simulink model "UnmilsElectrodeMapping"  (R2022b)
settings: Solver=VariableStepAuto  StartTime=0.0  StopTime=10.0  RelTol=1e-3
undefined symbols (not defined in the file or in its folder): ActFx, ActFy, ActFz, ActTx, ActTy, ActTz, dt, max_effort_V, min_effort_V, resolutionV, Ts_V
settings Model: Creator=ryankinzie  LastModifiedBy=ryankinzie

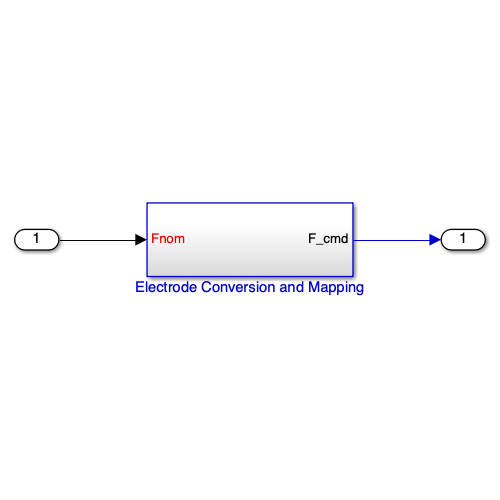
[thumbnail: Simulink's stored preview of the top-level diagram]
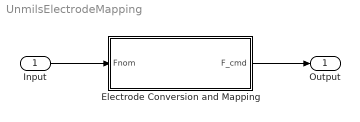
== system UnmilsElectrodeMapping ==
  Input : Inport
  Electrode Conversion and Mapping : Subsystem
  Output : Outport
  wires:
  Input/1 -> Electrode Conversion and Mapping/1(Fnom)
  Electrode Conversion and Mapping/1(F_cmd) -> Output/1

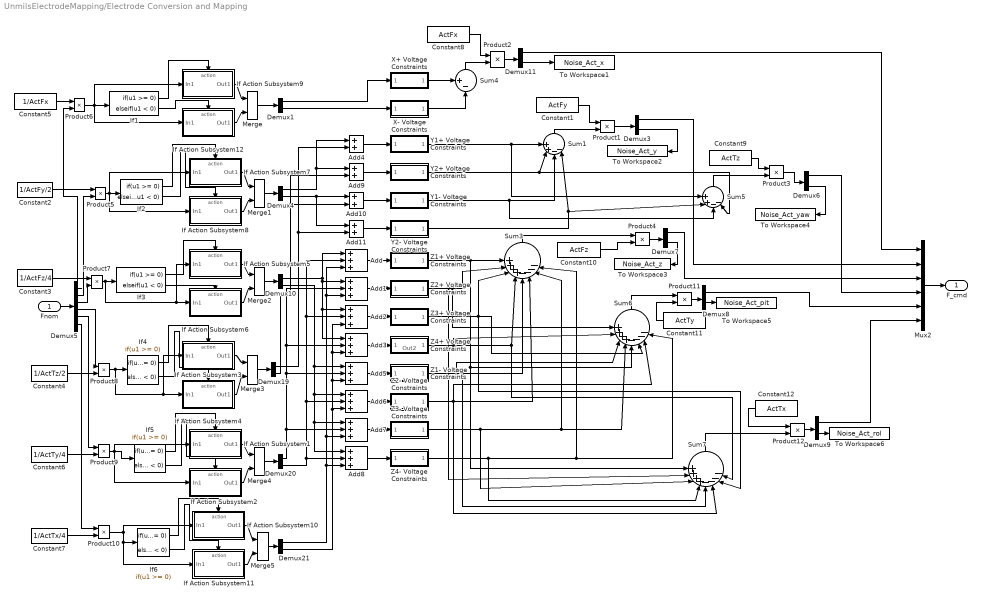
== system UnmilsElectrodeMapping/Electrode Conversion and Mapping ==
  Fnom : Inport
  Add{,1..3,5..8} (8 alike) : Sum  Inputs=+++
  Add{4,9..11} (4 alike) : Sum
  Constant1 : Constant  Value=ActFy
  Constant10 : Constant  Value=ActFz
  Constant11 : Constant  Value=ActTy
  Constant12 : Constant  Value=ActTx
  Constant2 : Constant  Value=1/ActFy/2
  Constant3 : Constant  Value=1/ActFz/4
  Constant4 : Constant  Value=1/ActTz/2
  Constant5 : Constant  Value=1/ActFx
  Constant6 : Constant  Value=1/ActTy/4
  Constant7 : Constant  Value=1/ActTx/4
  Constant8 : Constant  Value=ActFx
  Constant9 : Constant  Value=ActTz
  Demux{1,3..4,6..11,19..21} (12 alike) : Demux  Outputs=2
  Demux5 : Demux  Outputs=6
  If Action Subsystem1 : Subsystem  TreatAsAtomicUnit=on
  If Action Subsystem10 : Subsystem  TreatAsAtomicUnit=on
  If Action Subsystem11 : Subsystem  TreatAsAtomicUnit=on
  If Action Subsystem12 : Subsystem  TreatAsAtomicUnit=on
  If Action Subsystem2 : Subsystem  TreatAsAtomicUnit=on
  If Action Subsystem3 : Subsystem  TreatAsAtomicUnit=on
  If Action Subsystem4 : Subsystem  TreatAsAtomicUnit=on
  If Action Subsystem5 : Subsystem  TreatAsAtomicUnit=on
  If Action Subsystem6 : Subsystem  TreatAsAtomicUnit=on
  If Action Subsystem7 : Subsystem  TreatAsAtomicUnit=on
  If Action Subsystem8 : Subsystem  TreatAsAtomicUnit=on
  If Action Subsystem9 : Subsystem  TreatAsAtomicUnit=on
  If{1..6} (6 alike) : If  IfExpression=u1 >= 0  ElseIfExpressions=u1 < 0  ShowElse=off
  Merge{,1..5} (6 alike) : Merge
  Mux2 : Mux  Inputs=6
  Product{1..12} (12 alike) : Product
  Sum1 : Sum  Inputs=++--|
  Sum3 : Sum  Inputs=++++----|
  Sum4 : Sum  Inputs=+-|
  Sum5 : Sum  Inputs=++--|
  Sum6 : Sum  Inputs=++++----|
  Sum7 : Sum  Inputs=++++----|
  To Workspace1 : ToWorkspace  VariableName=Noise_Act_x  SaveFormat=Timeseries  SampleTime=-1
  To Workspace2 : ToWorkspace  VariableName=Noise_Act_y  SaveFormat=Timeseries  SampleTime=-1
  To Workspace3 : ToWorkspace  VariableName=Noise_Act_z  SaveFormat=Timeseries  SampleTime=-1
  To Workspace4 : ToWorkspace  VariableName=Noise_Act_yaw  SaveFormat=Timeseries  SampleTime=-1
  To Workspace5 : ToWorkspace  VariableName=Noise_Act_pit  SaveFormat=Timeseries  SampleTime=-1
  To Workspace6 : ToWorkspace  VariableName=Noise_Act_rol  SaveFormat=Timeseries  SampleTime=-1
  X+ Voltage Constraints : Subsystem
  X- Voltage Constraints : Subsystem
  Y1+ Voltage Constraints : Subsystem
  Y1- Voltage Constraints : Subsystem
  Y2+ Voltage Constraints : Subsystem
  Y2- Voltage Constraints : Subsystem
  Z1+ Voltage Constraints : Subsystem
  Z1- Voltage Constraints : Subsystem
  Z2+ Voltage Constraints : Subsystem
  Z2- Voltage Constraints : Subsystem
  Z3+ Voltage Constraints : Subsystem
  Z3- Voltage Constraints : Subsystem
  Z4+ Voltage Constraints : Subsystem
      settings: PortSchema="{\"entries\":[{\"content\":{\"sides\":[{\"content\":{\"connectorIds\":[\"In1\"]},\"type\":\"ConnectorPlacement.EquallySpacedRectSide\",\"uuid\":\"268a8257-2af5-491e-bd10-2121474e7c81\"},{\"content\":{\"connectorIds\":[\"Out1\"],\"side\":\"RIGHT\"},\"type\":\"ConnectorPlacement.EquallySpacedRectSide\",\"uuid\":\"02848540-b4c7-4bb5-8d33-e0a12813d580\"},{\"content\":{\"connectorIds\":[],\"side\":\"TOP\"},\"type\":\"ConnectorPlacement.EquallySpacedRectSide\",\"uuid\":\"923eb65b-e7e4-4c35-9b37-324be502522f\"},{\"content\":{\"connectorIds\":[\"Out2\"],\"side\":\"BOTTOM\"},\"type\":\"ConnectorPlacement.EquallySpacedRectSide\",\"uuid\":\"50220811-6f84-4747-b900-a7dc6eb7e9f2\"},{\"content\":{\"connectorIds\":[],\"side\":\"HIDDEN\"},\"type\":\"ConnectorPlacement.EquallySpacedRectSide\",\"uuid\":\"7f2e36bf-1a7e-4bb9-969e-4fa6a7ae6d46\"}]},\"type\":\"ConnectorPlacement.EquallySpacedConnector\",\"uuid\":\"5035f1e4-cb80-4656-b4e7-b23e8e10be7f\"}],\"packageUris\":[\"http://schema.mathworks.com/mf0/Connector/R2020b\"],\"version\":\"1.0\"}"
  Z4- Voltage Constraints : Subsystem
  F_cmd : Outport
  wires:
  Fnom/1 -> Demux5/1
  If Action Subsystem12/1(Out1) -> Merge/2
  Merge/1 -> Demux1/1
  If Action Subsystem9/1(Out1) -> Merge/1
  If1/2 -> If Action Subsystem12/Action
  If1/1 -> If Action Subsystem9/Action
  Demux1/1 -> X+ Voltage Constraints/1(Fnom)
  Merge1/1 -> Demux4/1
  If2/1 -> If Action Subsystem7/Action
  If2/2 -> If Action Subsystem8/Action
  If Action Subsystem8/1(Out1) -> Merge1/2
  If Action Subsystem7/1(Out1) -> Merge1/1
  If Action Subsystem6/1(Out1) -> Merge2/2
  If3/1 -> If Action Subsystem5/Action
  Merge2/1 -> Demux10/1
  If3/2 -> If Action Subsystem6/Action
  If Action Subsystem5/1(Out1) -> Merge2/1
  Z1+ Voltage Constraints/1(VOut) -> Sum7/1, Sum6/5, Sum3/1
  Z2+ Voltage Constraints/1(VOut) -> Sum3/2, Sum6/1, Sum7/2
  Z3+ Voltage Constraints/1(VOut) -> Sum7/7, Sum6/6, Sum3/3
  Z4+ Voltage Constraints/1(VOut) -> Sum7/8, Sum3/4, Sum6/2
  Z1- Voltage Constraints/1(VOut) -> Sum7/5, Sum3/5, Sum6/3
  Z2- Voltage Constraints/1(VOut) -> Sum7/6, Sum6/7, Sum3/6
  Z3- Voltage Constraints/1(VOut) -> Sum7/3, Sum6/4, Sum3/7
  Z4- Voltage Constraints/1(VOut) -> Sum6/8, Sum3/8, Sum7/4
  If4/2 -> If Action Subsystem4/Action
  If Action Subsystem3/1(Out1) -> Merge3/1
  If Action Subsystem4/1(Out1) -> Merge3/2
  If4/1 -> If Action Subsystem3/Action
  Merge3/1 -> Demux19/1
  Constant5/1 -> Product6/1
  Demux5/1 -> Product6/2
  Product6/1 -> If Action Subsystem12/1(In1), If Action Subsystem9/1(In1), If1/1
  Constant2/1 -> Product5/1
  Demux5/2 -> Product5/2
  Product5/1 -> If Action Subsystem8/1(In1), If Action Subsystem7/1(In1), If2/1
  Constant3/1 -> Product7/1
  Product7/1 -> If Action Subsystem5/1(In1), If Action Subsystem6/1(In1), If3/1
  Demux5/3 -> Product7/2
  Product8/1 -> If Action Subsystem3/1(In1), If Action Subsystem4/1(In1), If4/1
  Constant4/1 -> Product8/2
  Demux5/4 -> Product8/1
  Demux5/5 -> Product9/1
  Constant6/1 -> Product9/2
  Demux5/6 -> Product10/1
  Constant7/1 -> Product10/2
  Merge4/1 -> Demux20/1
  If5/1 -> If Action Subsystem1/Action
  If5/2 -> If Action Subsystem2/Action
  If Action Subsystem1/1(Out1) -> Merge4/1
  If Action Subsystem2/1(Out1) -> Merge4/2
  Product9/1 -> If Action Subsystem1/1(In1), If Action Subsystem2/1(In1), If5/1
  Merge5/1 -> Demux21/1
  If6/1 -> If Action Subsystem10/Action
  If6/2 -> If Action Subsystem11/Action
  If Action Subsystem10/1(Out1) -> Merge5/1
  If Action Subsystem11/1(Out1) -> Merge5/2
  Product10/1 -> If Action Subsystem10/1(In1), If Action Subsystem11/1(In1), If6/1
  Mux2/1 -> F_cmd/1
  Add/1 -> Z1+ Voltage Constraints/1(Fnom)
  Add1/1 -> Z2+ Voltage Constraints/1(Fnom)
  Add2/1 -> Z3+ Voltage Constraints/1(Fnom)
  Add3/1 -> Z4+ Voltage Constraints/1(Fnom)
  Demux10/2 -> Add5/1, Add6/1, Add7/1, Add8/1
  Add5/1 -> Z1- Voltage Constraints/1(Fnom)
  Add6/1 -> Z2- Voltage Constraints/1(Fnom)
  Add7/1 -> Z3- Voltage Constraints/1(Fnom)
  Add8/1 -> Z4- Voltage Constraints/1(Fnom)
  Demux10/1 -> Add3/1, Add2/1, Add1/1, Add/1
  Add4/1 -> Y1+ Voltage Constraints/1(Fnom)
  Add9/1 -> Y2+ Voltage Constraints/1(Fnom)
  Add10/1 -> Y1- Voltage Constraints/1(Fnom)
  Add11/1 -> Y2- Voltage Constraints/1(Fnom)
  Demux4/1 -> Add9/1, Add4/1
  Demux4/2 -> Add11/1, Add10/1
  Y1+ Voltage Constraints/1(VOut) -> Sum5/1, Sum1/1
  Y2+ Voltage Constraints/1(VOut) -> Sum5/4, Sum1/2
  Y1- Voltage Constraints/1(VOut) -> Sum5/3, Sum1/3
  Y2- Voltage Constraints/1(VOut) -> Sum5/2, Sum1/4
  Product1/1 -> Demux3/1
  Demux3/2 -> To Workspace2/1
  Demux3/1 -> Mux2/2
  Product3/1 -> Demux6/1
  Demux6/2 -> To Workspace4/1
  Demux6/1 -> Mux2/4
  Sum3/1 -> Product4/1
  Product4/1 -> Demux7/1
  Demux7/1 -> Mux2/3
  Demux7/2 -> To Workspace3/1
  Demux19/1 -> Add11/2, Add4/2
  Demux19/2 -> Add10/2, Add9/2
  Demux20/1 -> Add5/2, Add3/2, Add1/2, Add7/2
  Demux20/2 -> Add6/2, Add2/2, Add/2, Add8/2
  Demux21/1 -> Add1/3, Add/3, Add7/3, Add8/3
  Demux21/2 -> Add6/3, Add5/3, Add2/3, Add3/3
  Demux8/2 -> To Workspace5/1
  Demux8/1 -> Mux2/5
  Demux9/2 -> To Workspace6/1
  Demux9/1 -> Mux2/6
  X+ Voltage Constraints/1(Fout) -> Sum4/1
  Demux11/1 -> Mux2/1
  Constant1/1 -> Product1/1
  Sum1/1 -> Product1/2
  Constant8/1 -> Product2/1
  Constant9/1 -> Product3/1
  Sum5/1 -> Product3/2
  Constant10/1 -> Product4/2
  Product11/1 -> Demux8/1
  Constant11/1 -> Product11/2
  Sum6/1 -> Product11/1
  Constant12/1 -> Product12/1
  Product12/1 -> Demux9/1
  Sum7/1 -> Product12/2
  Demux11/2 -> To Workspace1/1
  Demux1/2 -> X- Voltage Constraints/1(Fnom)
  X- Voltage Constraints/1(Fout) -> Sum4/2
  Product2/1 -> Demux11/1
  Sum4/1 -> Product2/2

== system UnmilsElectrodeMapping/Electrode Conversion and Mapping/If Action Subsystem1 ==
  In1 : Inport
  Action Port : ActionPort
  Abs1 : Abs  SaturateOnIntegerOverflow=off
  Constant1 : Constant  Value=0
  Mux6 : Mux  Inputs=2
  Sqrt1 : Sqrt
  Out1 : Outport
  wires:
  In1/1 -> Abs1/1
  Mux6/1 -> Out1/1
  Constant1/1 -> Mux6/2
  Abs1/1 -> Sqrt1/1
  Sqrt1/1 -> Mux6/1

== system UnmilsElectrodeMapping/Electrode Conversion and Mapping/If Action Subsystem10 ==
  In1 : Inport
  Action Port : ActionPort
  Abs1 : Abs  SaturateOnIntegerOverflow=off
  Constant1 : Constant  Value=0
  Mux6 : Mux  Inputs=2
  Sqrt1 : Sqrt
  Out1 : Outport
  wires:
  In1/1 -> Abs1/1
  Mux6/1 -> Out1/1
  Constant1/1 -> Mux6/2
  Abs1/1 -> Sqrt1/1
  Sqrt1/1 -> Mux6/1

== system UnmilsElectrodeMapping/Electrode Conversion and Mapping/If Action Subsystem11 ==
  In1 : Inport
  Action Port : ActionPort
  Abs1 : Abs  SaturateOnIntegerOverflow=off
  Constant1 : Constant  Value=0
  Mux6 : Mux  Inputs=2
  Sqrt1 : Sqrt
  Out1 : Outport
  wires:
  In1/1 -> Abs1/1
  Mux6/1 -> Out1/1
  Constant1/1 -> Mux6/1
  Abs1/1 -> Sqrt1/1
  Sqrt1/1 -> Mux6/2

== system UnmilsElectrodeMapping/Electrode Conversion and Mapping/If Action Subsystem12 ==
  In1 : Inport
  Action Port : ActionPort
  Abs1 : Abs  SaturateOnIntegerOverflow=off
  Constant1 : Constant  Value=0
  Mux6 : Mux  Inputs=2
  Sqrt1 : Sqrt
  Out1 : Outport
  wires:
  In1/1 -> Abs1/1
  Mux6/1 -> Out1/1
  Constant1/1 -> Mux6/1
  Abs1/1 -> Sqrt1/1
  Sqrt1/1 -> Mux6/2

== system UnmilsElectrodeMapping/Electrode Conversion and Mapping/If Action Subsystem2 ==
  In1 : Inport
  Action Port : ActionPort
  Abs1 : Abs  SaturateOnIntegerOverflow=off
  Constant1 : Constant  Value=0
  Mux6 : Mux  Inputs=2
  Sqrt1 : Sqrt
  Out1 : Outport
  wires:
  In1/1 -> Abs1/1
  Mux6/1 -> Out1/1
  Constant1/1 -> Mux6/1
  Abs1/1 -> Sqrt1/1
  Sqrt1/1 -> Mux6/2

== system UnmilsElectrodeMapping/Electrode Conversion and Mapping/If Action Subsystem3 ==
  In1 : Inport
  Action Port : ActionPort
  Abs1 : Abs  SaturateOnIntegerOverflow=off
  Constant1 : Constant  Value=0
  Mux6 : Mux  Inputs=2
  Sqrt1 : Sqrt
  Out1 : Outport
  wires:
  In1/1 -> Abs1/1
  Mux6/1 -> Out1/1
  Constant1/1 -> Mux6/2
  Abs1/1 -> Sqrt1/1
  Sqrt1/1 -> Mux6/1

== system UnmilsElectrodeMapping/Electrode Conversion and Mapping/If Action Subsystem4 ==
  In1 : Inport
  Action Port : ActionPort
  Abs1 : Abs  SaturateOnIntegerOverflow=off
  Constant1 : Constant  Value=0
  Mux6 : Mux  Inputs=2
  Sqrt1 : Sqrt
  Out1 : Outport
  wires:
  In1/1 -> Abs1/1
  Mux6/1 -> Out1/1
  Constant1/1 -> Mux6/1
  Abs1/1 -> Sqrt1/1
  Sqrt1/1 -> Mux6/2

== system UnmilsElectrodeMapping/Electrode Conversion and Mapping/If Action Subsystem5 ==
  In1 : Inport
  Action Port : ActionPort
  Abs1 : Abs  SaturateOnIntegerOverflow=off
  Constant1 : Constant  Value=0
  Mux6 : Mux  Inputs=2
  Sqrt1 : Sqrt
  Out1 : Outport
  wires:
  In1/1 -> Abs1/1
  Mux6/1 -> Out1/1
  Constant1/1 -> Mux6/2
  Abs1/1 -> Sqrt1/1
  Sqrt1/1 -> Mux6/1

== system UnmilsElectrodeMapping/Electrode Conversion and Mapping/If Action Subsystem6 ==
  In1 : Inport
  Action Port : ActionPort
  Abs1 : Abs  SaturateOnIntegerOverflow=off
  Constant1 : Constant  Value=0
  Mux6 : Mux  Inputs=2
  Sqrt1 : Sqrt
  Out1 : Outport
  wires:
  In1/1 -> Abs1/1
  Mux6/1 -> Out1/1
  Constant1/1 -> Mux6/1
  Abs1/1 -> Sqrt1/1
  Sqrt1/1 -> Mux6/2

== system UnmilsElectrodeMapping/Electrode Conversion and Mapping/If Action Subsystem7 ==
  In1 : Inport
  Action Port : ActionPort
  Abs1 : Abs  SaturateOnIntegerOverflow=off
  Constant1 : Constant  Value=0
  Mux6 : Mux  Inputs=2
  Sqrt1 : Sqrt
  Out1 : Outport
  wires:
  In1/1 -> Abs1/1
  Mux6/1 -> Out1/1
  Constant1/1 -> Mux6/2
  Abs1/1 -> Sqrt1/1
  Sqrt1/1 -> Mux6/1

== system UnmilsElectrodeMapping/Electrode Conversion and Mapping/If Action Subsystem8 ==
  In1 : Inport
  Action Port : ActionPort
  Abs1 : Abs  SaturateOnIntegerOverflow=off
  Constant1 : Constant  Value=0
  Mux6 : Mux  Inputs=2
  Sqrt1 : Sqrt
  Out1 : Outport
  wires:
  In1/1 -> Abs1/1
  Mux6/1 -> Out1/1
  Constant1/1 -> Mux6/1
  Abs1/1 -> Sqrt1/1
  Sqrt1/1 -> Mux6/2

== system UnmilsElectrodeMapping/Electrode Conversion and Mapping/If Action Subsystem9 ==
  In1 : Inport
  Action Port : ActionPort
  Abs1 : Abs  SaturateOnIntegerOverflow=off
  Constant1 : Constant  Value=0
  Mux6 : Mux  Inputs=2
  Sqrt1 : Sqrt
  Out1 : Outport
  wires:
  In1/1 -> Abs1/1
  Mux6/1 -> Out1/1
  Constant1/1 -> Mux6/2
  Abs1/1 -> Sqrt1/1
  Sqrt1/1 -> Mux6/1

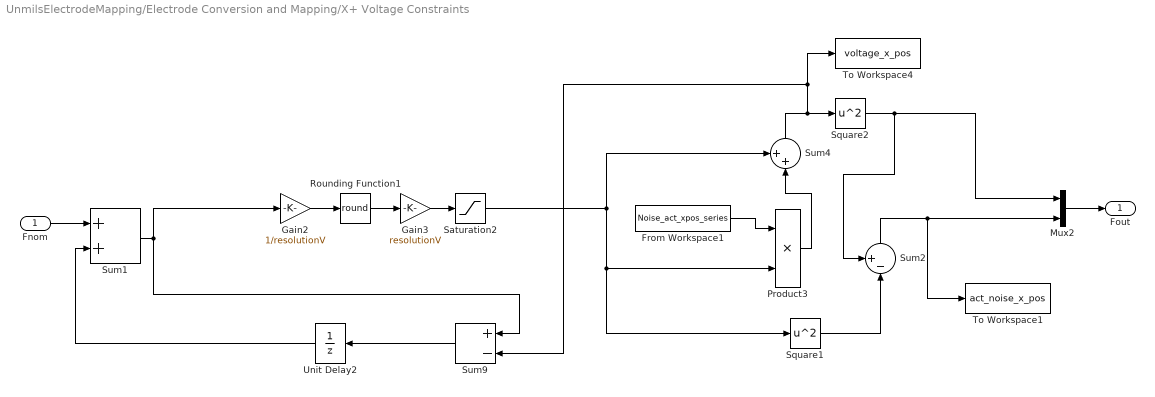
== system UnmilsElectrodeMapping/Electrode Conversion and Mapping/X+ Voltage Constraints ==
  Fnom : Inport
  From Workspace1 : FromWorkspace  VariableName=Noise_act_xpos_series  SampleTime=dt
  Gain2 : Gain  Gain=1/resolutionV
  Gain3 : Gain  Gain=resolutionV
  Mux2 : Mux  Inputs=2
  Product3 : Product
  Rounding Function1 : Rounding  Operator=round
  Saturation2 : Saturate  UpperLimit=max_effort_V  LowerLimit=min_effort_V  RndMeth=Round
  Square1 : Math  Operator=square
  Square2 : Math  Operator=square
  Sum1 : Sum  InputSameDT=on  SaturateOnIntegerOverflow=on  OutDataTypeStr=Inherit: Same as first input
  Sum2 : Sum  Inputs=+-|
  Sum4 : Sum  Inputs=++|
  Sum9 : Sum  Inputs=+-  InputSameDT=on  SaturateOnIntegerOverflow=on  OutDataTypeStr=Inherit: Same as first input
  To Workspace1 : ToWorkspace  VariableName=act_noise_x_pos  SaveFormat=Timeseries  SampleTime=-1
  To Workspace4 : ToWorkspace  VariableName=voltage_x_pos  SaveFormat=Timeseries  SampleTime=-1
  Unit Delay2 : UnitDelay  SampleTime=Ts_V  HasFrameUpgradeWarning=on
  Fout : Outport
  wires:
  Sum9/1 -> Unit Delay2/1
  Unit Delay2/1 -> Sum1/2
  Fnom/1 -> Sum1/1
  Gain2/1 -> Rounding Function1/1
  Gain3/1 -> Saturation2/1
  Rounding Function1/1 -> Gain3/1
  Sum1/1 -> Gain2/1, Sum9/1
  Saturation2/1 -> Product3/2, Square1/1, Sum4/1
  Product3/1 -> Sum4/2
  Mux2/1 -> Fout/1
  Square2/1 -> Sum2/1, Mux2/1
  Sum4/1 -> Sum9/2, To Workspace4/1, Square2/1
  Square1/1 -> Sum2/2
  Sum2/1 -> To Workspace1/1, Mux2/2
  From Workspace1/1 -> Product3/1

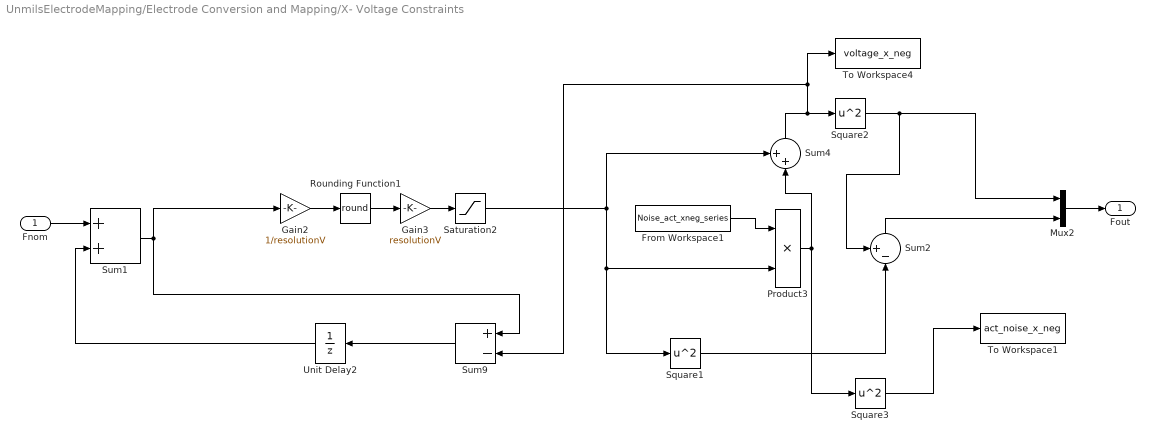
== system UnmilsElectrodeMapping/Electrode Conversion and Mapping/X- Voltage Constraints ==
  Fnom : Inport
  From Workspace1 : FromWorkspace  VariableName=Noise_act_xneg_series  SampleTime=dt
  Gain2 : Gain  Gain=1/resolutionV
  Gain3 : Gain  Gain=resolutionV
  Mux2 : Mux  Inputs=2
  Product3 : Product
  Rounding Function1 : Rounding  Operator=round
  Saturation2 : Saturate  UpperLimit=max_effort_V  LowerLimit=min_effort_V  RndMeth=Round
  Square1 : Math  Operator=square
  Square2 : Math  Operator=square
  Square3 : Math  Operator=square
  Sum1 : Sum  InputSameDT=on  SaturateOnIntegerOverflow=on  OutDataTypeStr=Inherit: Same as first input
  Sum2 : Sum  Inputs=+-|
  Sum4 : Sum  Inputs=++|
  Sum9 : Sum  Inputs=+-  InputSameDT=on  SaturateOnIntegerOverflow=on  OutDataTypeStr=Inherit: Same as first input
  To Workspace1 : ToWorkspace  VariableName=act_noise_x_neg  SaveFormat=Timeseries  SampleTime=-1
  To Workspace4 : ToWorkspace  VariableName=voltage_x_neg  SaveFormat=Timeseries  SampleTime=-1
  Unit Delay2 : UnitDelay  SampleTime=Ts_V  HasFrameUpgradeWarning=on
  Fout : Outport
  wires:
  Sum9/1 -> Unit Delay2/1
  Unit Delay2/1 -> Sum1/2
  Fnom/1 -> Sum1/1
  Gain2/1 -> Rounding Function1/1
  Gain3/1 -> Saturation2/1
  Rounding Function1/1 -> Gain3/1
  Sum1/1 -> Gain2/1, Sum9/1
  Product3/1 -> Square3/1, Sum4/2
  Mux2/1 -> Fout/1
  Square2/1 -> Mux2/1, Sum2/1
  Sum4/1 -> Sum9/2, To Workspace4/1, Square2/1
  Square1/1 -> Sum2/2
  Sum2/1 -> Mux2/2
  Saturation2/1 -> Product3/2, Square1/1, Sum4/1
  From Workspace1/1 -> Product3/1
  Square3/1 -> To Workspace1/1

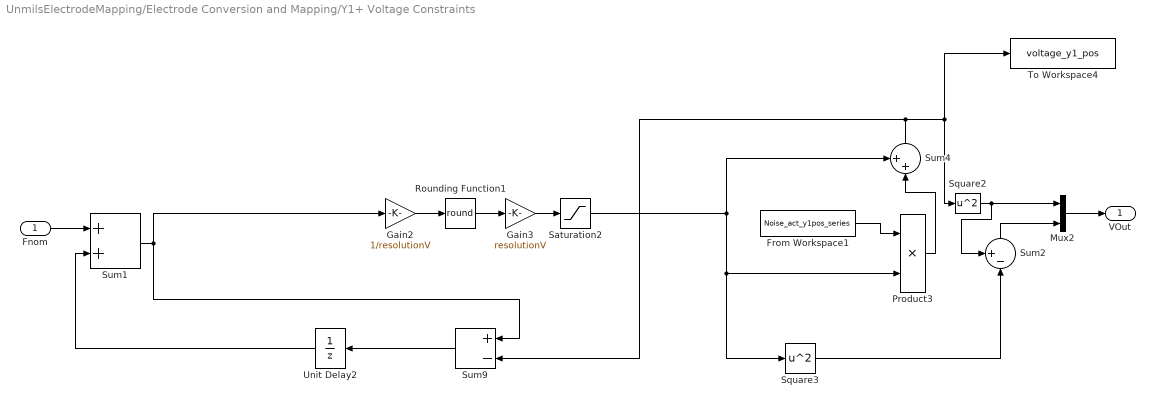
== system UnmilsElectrodeMapping/Electrode Conversion and Mapping/Y1+ Voltage Constraints ==
  Fnom : Inport
  From Workspace1 : FromWorkspace  VariableName=Noise_act_y1pos_series  SampleTime=dt
  Gain2 : Gain  Gain=1/resolutionV
  Gain3 : Gain  Gain=resolutionV
  Mux2 : Mux  Inputs=2
  Product3 : Product
  Rounding Function1 : Rounding  Operator=round
  Saturation2 : Saturate  UpperLimit=max_effort_V  LowerLimit=min_effort_V  RndMeth=Round
  Square2 : Math  Operator=square
  Square3 : Math  Operator=square
  Sum1 : Sum  InputSameDT=on  SaturateOnIntegerOverflow=on  OutDataTypeStr=Inherit: Same as first input
  Sum2 : Sum  Inputs=+-|
  Sum4 : Sum  Inputs=++|
  Sum9 : Sum  Inputs=+-  InputSameDT=on  SaturateOnIntegerOverflow=on  OutDataTypeStr=Inherit: Same as first input
  To Workspace4 : ToWorkspace  VariableName=voltage_y1_pos  SaveFormat=Timeseries  SampleTime=-1
  Unit Delay2 : UnitDelay  SampleTime=Ts_V  HasFrameUpgradeWarning=on
  VOut : Outport
  wires:
  Sum9/1 -> Unit Delay2/1
  Unit Delay2/1 -> Sum1/2
  Fnom/1 -> Sum1/1
  Gain2/1 -> Rounding Function1/1
  Gain3/1 -> Saturation2/1
  Rounding Function1/1 -> Gain3/1
  Sum1/1 -> Gain2/1, Sum9/1
  Mux2/1 -> VOut/1
  Sum4/1 -> To Workspace4/1, Square2/1, Sum9/2
  Square2/1 -> Sum2/1, Mux2/1
  Sum2/1 -> Mux2/2
  Square3/1 -> Sum2/2
  Saturation2/1 -> Product3/2, Square3/1, Sum4/1
  From Workspace1/1 -> Product3/1
  Product3/1 -> Sum4/2

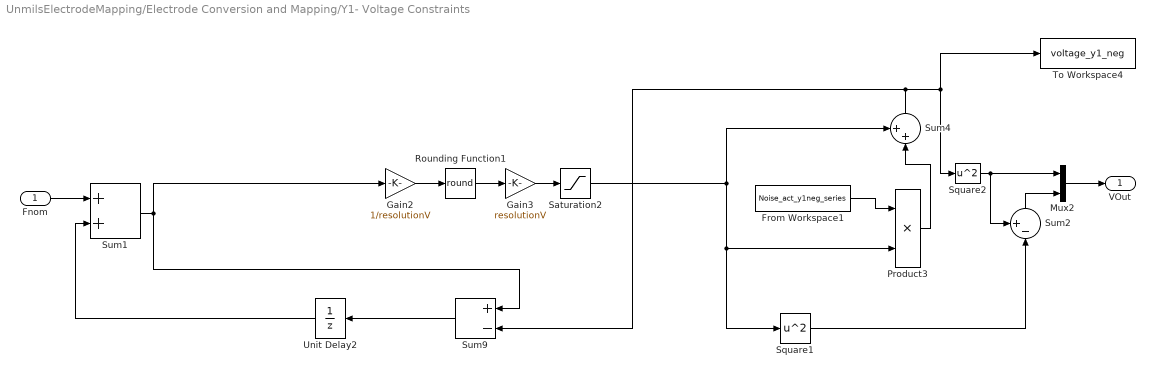
== system UnmilsElectrodeMapping/Electrode Conversion and Mapping/Y1- Voltage Constraints ==
  Fnom : Inport
  From Workspace1 : FromWorkspace  VariableName=Noise_act_y1neg_series  SampleTime=dt
  Gain2 : Gain  Gain=1/resolutionV
  Gain3 : Gain  Gain=resolutionV
  Mux2 : Mux  Inputs=2
  Product3 : Product
  Rounding Function1 : Rounding  Operator=round
  Saturation2 : Saturate  UpperLimit=max_effort_V  LowerLimit=min_effort_V  RndMeth=Round
  Square1 : Math  Operator=square
  Square2 : Math  Operator=square
  Sum1 : Sum  InputSameDT=on  SaturateOnIntegerOverflow=on  OutDataTypeStr=Inherit: Same as first input
  Sum2 : Sum  Inputs=+-|
  Sum4 : Sum  Inputs=++|
  Sum9 : Sum  Inputs=+-  InputSameDT=on  SaturateOnIntegerOverflow=on  OutDataTypeStr=Inherit: Same as first input
  To Workspace4 : ToWorkspace  VariableName=voltage_y1_neg  SaveFormat=Timeseries  SampleTime=-1
  Unit Delay2 : UnitDelay  SampleTime=Ts_V  HasFrameUpgradeWarning=on
  VOut : Outport
  wires:
  Sum9/1 -> Unit Delay2/1
  Unit Delay2/1 -> Sum1/2
  Fnom/1 -> Sum1/1
  Gain2/1 -> Rounding Function1/1
  Gain3/1 -> Saturation2/1
  Rounding Function1/1 -> Gain3/1
  Sum1/1 -> Gain2/1, Sum9/1
  Mux2/1 -> VOut/1
  Square2/1 -> Sum2/1, Mux2/1
  Sum4/1 -> To Workspace4/1, Square2/1, Sum9/2
  Square1/1 -> Sum2/2
  Sum2/1 -> Mux2/2
  Saturation2/1 -> Product3/2, Square1/1, Sum4/1
  From Workspace1/1 -> Product3/1
  Product3/1 -> Sum4/2

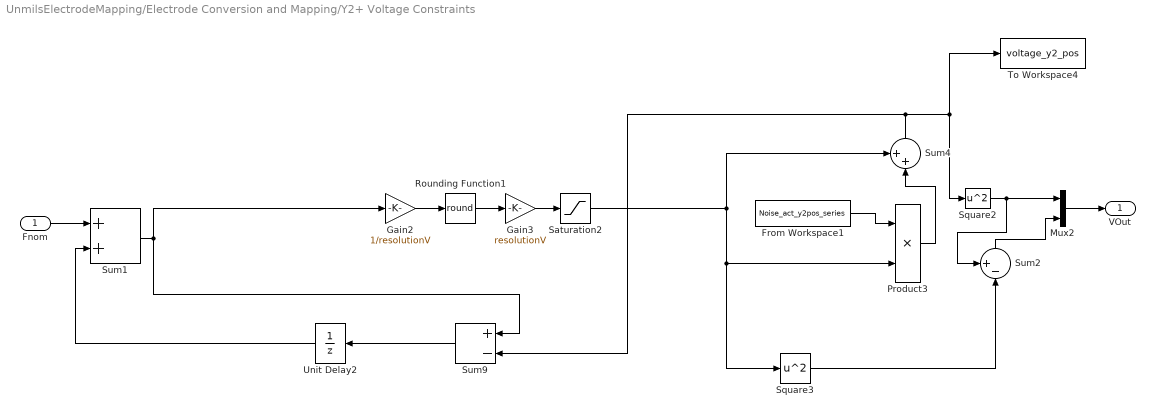
== system UnmilsElectrodeMapping/Electrode Conversion and Mapping/Y2+ Voltage Constraints ==
  Fnom : Inport
  From Workspace1 : FromWorkspace  VariableName=Noise_act_y2pos_series  SampleTime=dt
  Gain2 : Gain  Gain=1/resolutionV
  Gain3 : Gain  Gain=resolutionV
  Mux2 : Mux  Inputs=2
  Product3 : Product
  Rounding Function1 : Rounding  Operator=round
  Saturation2 : Saturate  UpperLimit=max_effort_V  LowerLimit=min_effort_V  RndMeth=Round
  Square2 : Math  Operator=square
  Square3 : Math  Operator=square
  Sum1 : Sum  InputSameDT=on  SaturateOnIntegerOverflow=on  OutDataTypeStr=Inherit: Same as first input
  Sum2 : Sum  Inputs=+-|
  Sum4 : Sum  Inputs=++|
  Sum9 : Sum  Inputs=+-  InputSameDT=on  SaturateOnIntegerOverflow=on  OutDataTypeStr=Inherit: Same as first input
  To Workspace4 : ToWorkspace  VariableName=voltage_y2_pos  SaveFormat=Timeseries  SampleTime=-1
  Unit Delay2 : UnitDelay  SampleTime=Ts_V  HasFrameUpgradeWarning=on
  VOut : Outport
  wires:
  Sum9/1 -> Unit Delay2/1
  Unit Delay2/1 -> Sum1/2
  Fnom/1 -> Sum1/1
  Gain2/1 -> Rounding Function1/1
  Gain3/1 -> Saturation2/1
  Rounding Function1/1 -> Gain3/1
  Sum1/1 -> Gain2/1, Sum9/1
  Mux2/1 -> VOut/1
  Square2/1 -> Sum2/1, Mux2/1
  Sum4/1 -> To Workspace4/1, Square2/1, Sum9/2
  Square3/1 -> Sum2/2
  Sum2/1 -> Mux2/2
  Saturation2/1 -> Product3/2, Square3/1, Sum4/1
  From Workspace1/1 -> Product3/1
  Product3/1 -> Sum4/2

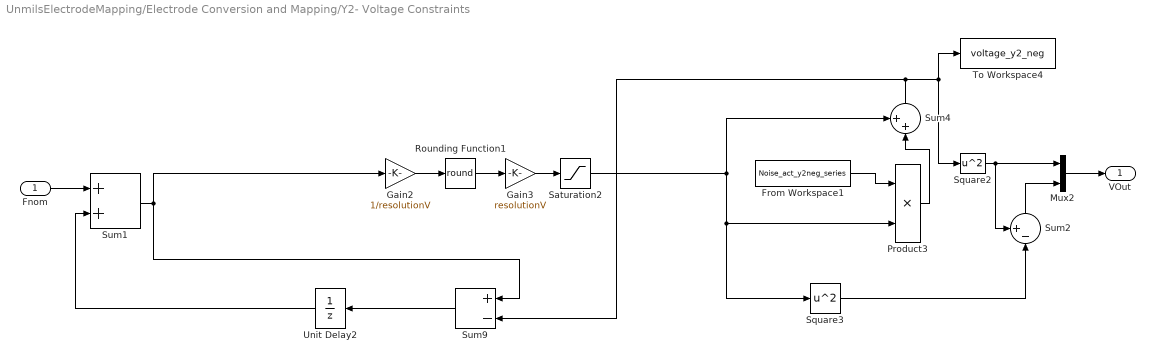
== system UnmilsElectrodeMapping/Electrode Conversion and Mapping/Y2- Voltage Constraints ==
  Fnom : Inport
  From Workspace1 : FromWorkspace  VariableName=Noise_act_y2neg_series  SampleTime=dt
  Gain2 : Gain  Gain=1/resolutionV
  Gain3 : Gain  Gain=resolutionV
  Mux2 : Mux  Inputs=2
  Product3 : Product
  Rounding Function1 : Rounding  Operator=round
  Saturation2 : Saturate  UpperLimit=max_effort_V  LowerLimit=min_effort_V  RndMeth=Round
  Square2 : Math  Operator=square
  Square3 : Math  Operator=square
  Sum1 : Sum  InputSameDT=on  SaturateOnIntegerOverflow=on  OutDataTypeStr=Inherit: Same as first input
  Sum2 : Sum  Inputs=+-|
  Sum4 : Sum  Inputs=++|
  Sum9 : Sum  Inputs=+-  InputSameDT=on  SaturateOnIntegerOverflow=on  OutDataTypeStr=Inherit: Same as first input
  To Workspace4 : ToWorkspace  VariableName=voltage_y2_neg  SaveFormat=Timeseries  SampleTime=-1
  Unit Delay2 : UnitDelay  SampleTime=Ts_V  HasFrameUpgradeWarning=on
  VOut : Outport
  wires:
  Sum9/1 -> Unit Delay2/1
  Unit Delay2/1 -> Sum1/2
  Fnom/1 -> Sum1/1
  Gain2/1 -> Rounding Function1/1
  Gain3/1 -> Saturation2/1
  Rounding Function1/1 -> Gain3/1
  Sum1/1 -> Gain2/1, Sum9/1
  Mux2/1 -> VOut/1
  Square2/1 -> Sum2/1, Mux2/1
  Sum4/1 -> To Workspace4/1, Square2/1, Sum9/2
  Square3/1 -> Sum2/2
  Sum2/1 -> Mux2/2
  Saturation2/1 -> Product3/2, Square3/1, Sum4/1
  From Workspace1/1 -> Product3/1
  Product3/1 -> Sum4/2

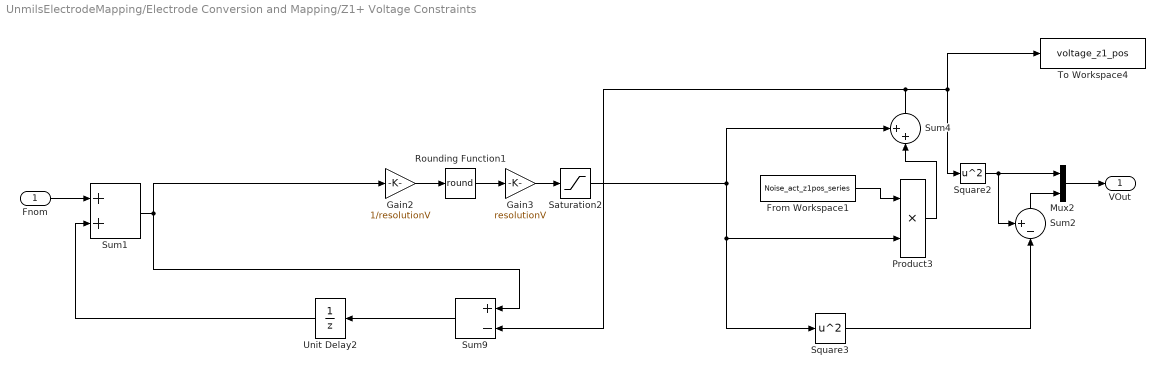
== system UnmilsElectrodeMapping/Electrode Conversion and Mapping/Z1+ Voltage Constraints ==
  Fnom : Inport
  From Workspace1 : FromWorkspace  VariableName=Noise_act_z1pos_series  SampleTime=dt
  Gain2 : Gain  Gain=1/resolutionV
  Gain3 : Gain  Gain=resolutionV
  Mux2 : Mux  Inputs=2
  Product3 : Product
  Rounding Function1 : Rounding  Operator=round
  Saturation2 : Saturate  UpperLimit=max_effort_V  LowerLimit=min_effort_V  RndMeth=Round
  Square2 : Math  Operator=square
  Square3 : Math  Operator=square
  Sum1 : Sum  InputSameDT=on  SaturateOnIntegerOverflow=on  OutDataTypeStr=Inherit: Same as first input
  Sum2 : Sum  Inputs=+-|
  Sum4 : Sum  Inputs=++|
  Sum9 : Sum  Inputs=+-  InputSameDT=on  SaturateOnIntegerOverflow=on  OutDataTypeStr=Inherit: Same as first input
  To Workspace4 : ToWorkspace  VariableName=voltage_z1_pos  SaveFormat=Timeseries  SampleTime=-1
  Unit Delay2 : UnitDelay  SampleTime=Ts_V  HasFrameUpgradeWarning=on
  VOut : Outport
  wires:
  Sum9/1 -> Unit Delay2/1
  Unit Delay2/1 -> Sum1/2
  Fnom/1 -> Sum1/1
  Gain2/1 -> Rounding Function1/1
  Gain3/1 -> Saturation2/1
  Rounding Function1/1 -> Gain3/1
  Sum1/1 -> Gain2/1, Sum9/1
  Mux2/1 -> VOut/1
  Square2/1 -> Sum2/1, Mux2/1
  Sum4/1 -> To Workspace4/1, Square2/1, Sum9/2
  Square3/1 -> Sum2/2
  Sum2/1 -> Mux2/2
  Saturation2/1 -> Product3/2, Square3/1, Sum4/1
  From Workspace1/1 -> Product3/1
  Product3/1 -> Sum4/2

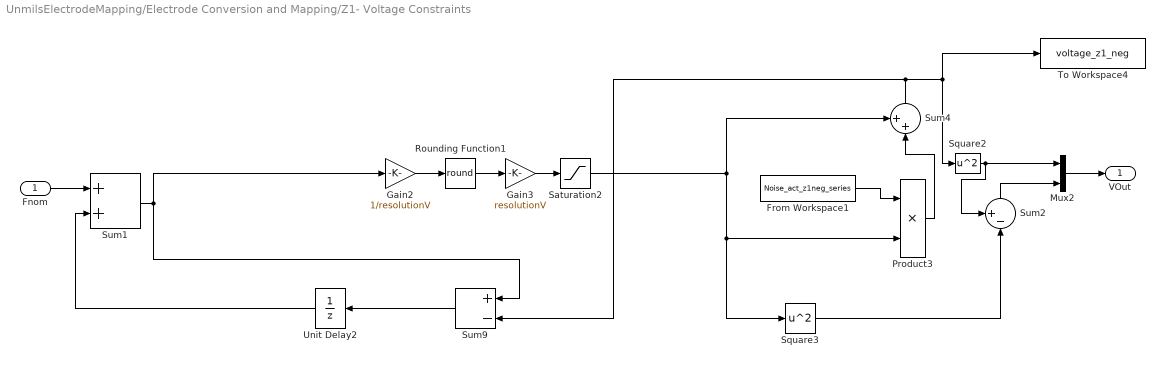
== system UnmilsElectrodeMapping/Electrode Conversion and Mapping/Z1- Voltage Constraints ==
  Fnom : Inport
  From Workspace1 : FromWorkspace  VariableName=Noise_act_z1neg_series  SampleTime=dt
  Gain2 : Gain  Gain=1/resolutionV
  Gain3 : Gain  Gain=resolutionV
  Mux2 : Mux  Inputs=2
  Product3 : Product
  Rounding Function1 : Rounding  Operator=round
  Saturation2 : Saturate  UpperLimit=max_effort_V  LowerLimit=min_effort_V  RndMeth=Round
  Square2 : Math  Operator=square
  Square3 : Math  Operator=square
  Sum1 : Sum  InputSameDT=on  SaturateOnIntegerOverflow=on  OutDataTypeStr=Inherit: Same as first input
  Sum2 : Sum  Inputs=+-|
  Sum4 : Sum  Inputs=++|
  Sum9 : Sum  Inputs=+-  InputSameDT=on  SaturateOnIntegerOverflow=on  OutDataTypeStr=Inherit: Same as first input
  To Workspace4 : ToWorkspace  VariableName=voltage_z1_neg  SaveFormat=Timeseries  SampleTime=-1
  Unit Delay2 : UnitDelay  SampleTime=Ts_V  HasFrameUpgradeWarning=on
  VOut : Outport
  wires:
  Sum9/1 -> Unit Delay2/1
  Unit Delay2/1 -> Sum1/2
  Fnom/1 -> Sum1/1
  Gain2/1 -> Rounding Function1/1
  Gain3/1 -> Saturation2/1
  Rounding Function1/1 -> Gain3/1
  Sum1/1 -> Gain2/1, Sum9/1
  Mux2/1 -> VOut/1
  Square2/1 -> Sum2/1, Mux2/1
  Sum4/1 -> To Workspace4/1, Square2/1, Sum9/2
  Square3/1 -> Sum2/2
  Sum2/1 -> Mux2/2
  Saturation2/1 -> Product3/2, Square3/1, Sum4/1
  From Workspace1/1 -> Product3/1
  Product3/1 -> Sum4/2

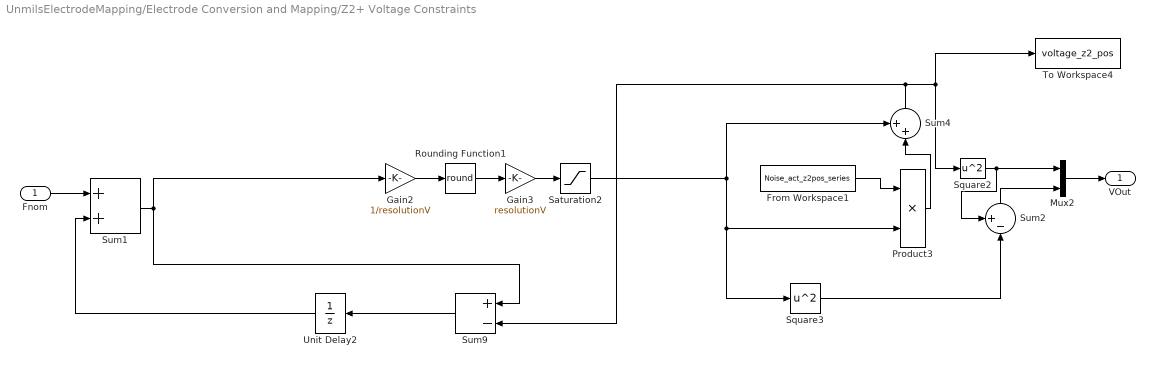
== system UnmilsElectrodeMapping/Electrode Conversion and Mapping/Z2+ Voltage Constraints ==
  Fnom : Inport
  From Workspace1 : FromWorkspace  VariableName=Noise_act_z2pos_series  SampleTime=dt
  Gain2 : Gain  Gain=1/resolutionV
  Gain3 : Gain  Gain=resolutionV
  Mux2 : Mux  Inputs=2
  Product3 : Product
  Rounding Function1 : Rounding  Operator=round
  Saturation2 : Saturate  UpperLimit=max_effort_V  LowerLimit=min_effort_V  RndMeth=Round
  Square2 : Math  Operator=square
  Square3 : Math  Operator=square
  Sum1 : Sum  InputSameDT=on  SaturateOnIntegerOverflow=on  OutDataTypeStr=Inherit: Same as first input
  Sum2 : Sum  Inputs=+-|
  Sum4 : Sum  Inputs=++|
  Sum9 : Sum  Inputs=+-  InputSameDT=on  SaturateOnIntegerOverflow=on  OutDataTypeStr=Inherit: Same as first input
  To Workspace4 : ToWorkspace  VariableName=voltage_z2_pos  SaveFormat=Timeseries  SampleTime=-1
  Unit Delay2 : UnitDelay  SampleTime=Ts_V  HasFrameUpgradeWarning=on
  VOut : Outport
  wires:
  Sum9/1 -> Unit Delay2/1
  Unit Delay2/1 -> Sum1/2
  Fnom/1 -> Sum1/1
  Gain2/1 -> Rounding Function1/1
  Gain3/1 -> Saturation2/1
  Rounding Function1/1 -> Gain3/1
  Sum1/1 -> Gain2/1, Sum9/1
  Mux2/1 -> VOut/1
  Square2/1 -> Sum2/1, Mux2/1
  Sum4/1 -> Square2/1, To Workspace4/1, Sum9/2
  Square3/1 -> Sum2/2
  Sum2/1 -> Mux2/2
  Saturation2/1 -> Product3/2, Square3/1, Sum4/1
  From Workspace1/1 -> Product3/1
  Product3/1 -> Sum4/2

== system UnmilsElectrodeMapping/Electrode Conversion and Mapping/Z2- Voltage Constraints ==
  Fnom : Inport
  From Workspace1 : FromWorkspace  VariableName=Noise_act_z2neg_series  SampleTime=dt
  Gain2 : Gain  Gain=1/resolutionV
  Gain3 : Gain  Gain=resolutionV
  Mux2 : Mux  Inputs=2
  Product3 : Product
  Rounding Function1 : Rounding  Operator=round
  Saturation2 : Saturate  UpperLimit=max_effort_V  LowerLimit=min_effort_V  RndMeth=Round
  Square2 : Math  Operator=square
  Square3 : Math  Operator=square
  Sum1 : Sum  InputSameDT=on  SaturateOnIntegerOverflow=on  OutDataTypeStr=Inherit: Same as first input
  Sum2 : Sum  Inputs=+-|
  Sum4 : Sum  Inputs=++|
  Sum9 : Sum  Inputs=+-  InputSameDT=on  SaturateOnIntegerOverflow=on  OutDataTypeStr=Inherit: Same as first input
  To Workspace4 : ToWorkspace  VariableName=voltage_z2_neg  SaveFormat=Timeseries  SampleTime=-1
  Unit Delay2 : UnitDelay  SampleTime=Ts_V  HasFrameUpgradeWarning=on
  VOut : Outport
  wires:
  Sum9/1 -> Unit Delay2/1
  Unit Delay2/1 -> Sum1/2
  Fnom/1 -> Sum1/1
  Gain2/1 -> Rounding Function1/1
  Gain3/1 -> Saturation2/1
  Rounding Function1/1 -> Gain3/1
  Sum1/1 -> Gain2/1, Sum9/1
  Mux2/1 -> VOut/1
  Square2/1 -> Sum2/1, Mux2/1
  Sum4/1 -> To Workspace4/1, Square2/1, Sum9/2
  Square3/1 -> Sum2/2
  Sum2/1 -> Mux2/2
  Saturation2/1 -> Product3/2, Square3/1, Sum4/1
  From Workspace1/1 -> Product3/1
  Product3/1 -> Sum4/2

== system UnmilsElectrodeMapping/Electrode Conversion and Mapping/Z3+ Voltage Constraints ==
  Fnom : Inport
  From Workspace1 : FromWorkspace  VariableName=Noise_act_z3pos_series  SampleTime=dt
  Gain2 : Gain  Gain=1/resolutionV
  Gain3 : Gain  Gain=resolutionV
  Mux2 : Mux  Inputs=2
  Product3 : Product
  Rounding Function1 : Rounding  Operator=round
  Saturation2 : Saturate  UpperLimit=max_effort_V  LowerLimit=min_effort_V  RndMeth=Round
  Square2 : Math  Operator=square
  Square3 : Math  Operator=square
  Sum1 : Sum  InputSameDT=on  SaturateOnIntegerOverflow=on  OutDataTypeStr=Inherit: Same as first input
  Sum2 : Sum  Inputs=+-|
  Sum4 : Sum  Inputs=++|
  Sum9 : Sum  Inputs=+-  InputSameDT=on  SaturateOnIntegerOverflow=on  OutDataTypeStr=Inherit: Same as first input
  To Workspace4 : ToWorkspace  VariableName=voltage_z3_pos  SaveFormat=Timeseries  SampleTime=-1
  Unit Delay2 : UnitDelay  SampleTime=Ts_V  HasFrameUpgradeWarning=on
  VOut : Outport
  wires:
  Sum9/1 -> Unit Delay2/1
  Unit Delay2/1 -> Sum1/2
  Fnom/1 -> Sum1/1
  Gain2/1 -> Rounding Function1/1
  Gain3/1 -> Saturation2/1
  Rounding Function1/1 -> Gain3/1
  Sum1/1 -> Gain2/1, Sum9/1
  Mux2/1 -> VOut/1
  Square2/1 -> Sum2/1, Mux2/1
  Sum4/1 -> To Workspace4/1, Square2/1, Sum9/2
  Square3/1 -> Sum2/2
  Sum2/1 -> Mux2/2
  Saturation2/1 -> Product3/2, Square3/1, Sum4/1
  From Workspace1/1 -> Product3/1
  Product3/1 -> Sum4/2

== system UnmilsElectrodeMapping/Electrode Conversion and Mapping/Z3- Voltage Constraints ==
  Fnom : Inport
  From Workspace1 : FromWorkspace  VariableName=Noise_act_z3neg_series  SampleTime=dt
  Gain2 : Gain  Gain=1/resolutionV
  Gain3 : Gain  Gain=resolutionV
  Mux2 : Mux  Inputs=2
  Product3 : Product
  Rounding Function1 : Rounding  Operator=round
  Saturation2 : Saturate  UpperLimit=max_effort_V  LowerLimit=min_effort_V  RndMeth=Round
  Square2 : Math  Operator=square
  Square3 : Math  Operator=square
  Sum1 : Sum  InputSameDT=on  SaturateOnIntegerOverflow=on  OutDataTypeStr=Inherit: Same as first input
  Sum2 : Sum  Inputs=+-|
  Sum4 : Sum  Inputs=++|
  Sum9 : Sum  Inputs=+-  InputSameDT=on  SaturateOnIntegerOverflow=on  OutDataTypeStr=Inherit: Same as first input
  To Workspace4 : ToWorkspace  VariableName=voltage_z3_neg  SaveFormat=Timeseries  SampleTime=-1
  Unit Delay2 : UnitDelay  SampleTime=Ts_V  HasFrameUpgradeWarning=on
  VOut : Outport
  wires:
  Sum9/1 -> Unit Delay2/1
  Unit Delay2/1 -> Sum1/2
  Fnom/1 -> Sum1/1
  Gain2/1 -> Rounding Function1/1
  Gain3/1 -> Saturation2/1
  Rounding Function1/1 -> Gain3/1
  Sum1/1 -> Gain2/1, Sum9/1
  Mux2/1 -> VOut/1
  Square2/1 -> Sum2/1, Mux2/1
  Sum4/1 -> To Workspace4/1, Square2/1, Sum9/2
  Square3/1 -> Sum2/2
  Sum2/1 -> Mux2/2
  Saturation2/1 -> Product3/2, Square3/1, Sum4/1
  From Workspace1/1 -> Product3/1
  Product3/1 -> Sum4/2

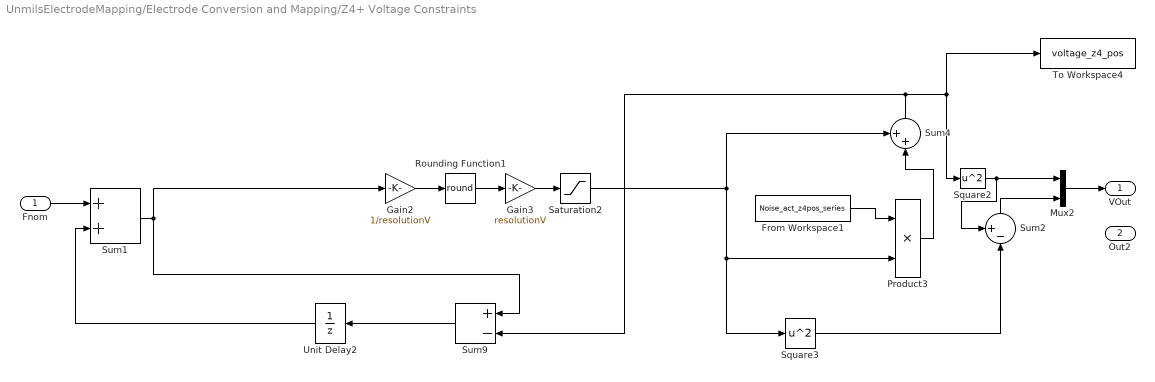
== system UnmilsElectrodeMapping/Electrode Conversion and Mapping/Z4+ Voltage Constraints ==
  Fnom : Inport
  From Workspace1 : FromWorkspace  VariableName=Noise_act_z4pos_series  SampleTime=dt
  Gain2 : Gain  Gain=1/resolutionV
  Gain3 : Gain  Gain=resolutionV
  Mux2 : Mux  Inputs=2
  Product3 : Product
  Rounding Function1 : Rounding  Operator=round
  Saturation2 : Saturate  UpperLimit=max_effort_V  LowerLimit=min_effort_V  RndMeth=Round
  Square2 : Math  Operator=square
  Square3 : Math  Operator=square
  Sum1 : Sum  InputSameDT=on  SaturateOnIntegerOverflow=on  OutDataTypeStr=Inherit: Same as first input
  Sum2 : Sum  Inputs=+-|
  Sum4 : Sum  Inputs=++|
  Sum9 : Sum  Inputs=+-  InputSameDT=on  SaturateOnIntegerOverflow=on  OutDataTypeStr=Inherit: Same as first input
  To Workspace4 : ToWorkspace  VariableName=voltage_z4_pos  SaveFormat=Timeseries  SampleTime=-1
  Unit Delay2 : UnitDelay  SampleTime=Ts_V  HasFrameUpgradeWarning=on
  VOut : Outport
  Out2 : Outport  Port=2
  wires:
  Sum9/1 -> Unit Delay2/1
  Unit Delay2/1 -> Sum1/2
  Fnom/1 -> Sum1/1
  Gain2/1 -> Rounding Function1/1
  Gain3/1 -> Saturation2/1
  Rounding Function1/1 -> Gain3/1
  Sum1/1 -> Gain2/1, Sum9/1
  Mux2/1 -> VOut/1
  Square2/1 -> Sum2/1, Mux2/1
  Sum4/1 -> To Workspace4/1, Square2/1, Sum9/2
  Square3/1 -> Sum2/2
  Sum2/1 -> Mux2/2
  Saturation2/1 -> Product3/2, Square3/1, Sum4/1
  From Workspace1/1 -> Product3/1
  Product3/1 -> Sum4/2

== system UnmilsElectrodeMapping/Electrode Conversion and Mapping/Z4- Voltage Constraints ==
  Fnom : Inport
  From Workspace1 : FromWorkspace  VariableName=Noise_act_z4neg_series  SampleTime=dt
  Gain2 : Gain  Gain=1/resolutionV
  Gain3 : Gain  Gain=resolutionV
  Mux2 : Mux  Inputs=2
  Product3 : Product
  Rounding Function1 : Rounding  Operator=round
  Saturation2 : Saturate  UpperLimit=max_effort_V  LowerLimit=min_effort_V  RndMeth=Round
  Square2 : Math  Operator=square
  Square3 : Math  Operator=square
  Sum1 : Sum  InputSameDT=on  SaturateOnIntegerOverflow=on  OutDataTypeStr=Inherit: Same as first input
  Sum2 : Sum  Inputs=+-|
  Sum4 : Sum  Inputs=++|
  Sum9 : Sum  Inputs=+-  InputSameDT=on  SaturateOnIntegerOverflow=on  OutDataTypeStr=Inherit: Same as first input
  To Workspace4 : ToWorkspace  VariableName=voltage_z4_neg  SaveFormat=Timeseries  SampleTime=-1
  Unit Delay2 : UnitDelay  SampleTime=Ts_V  HasFrameUpgradeWarning=on
  VOut : Outport
  wires:
  Sum9/1 -> Unit Delay2/1
  Unit Delay2/1 -> Sum1/2
  Fnom/1 -> Sum1/1
  Gain2/1 -> Rounding Function1/1
  Gain3/1 -> Saturation2/1
  Rounding Function1/1 -> Gain3/1
  Sum1/1 -> Gain2/1, Sum9/1
  Mux2/1 -> VOut/1
  Square2/1 -> Sum2/1, Mux2/1
  Sum4/1 -> To Workspace4/1, Square2/1, Sum9/2
  Square3/1 -> Sum2/2
  Sum2/1 -> Mux2/2
  Saturation2/1 -> Product3/2, Square3/1, Sum4/1
  From Workspace1/1 -> Product3/1
  Product3/1 -> Sum4/2
